simulink model "Controlador_PID_discreto"  (R2021a)
settings: Solver=VariableStepAuto  StartTime=0.0  StopTime=10.0  RelTol=1e-3
undefined symbols (not defined in the file): ba, ksa, ksia, ts
settings Model: Creator=fhlla  LastModifiedBy=fhlla

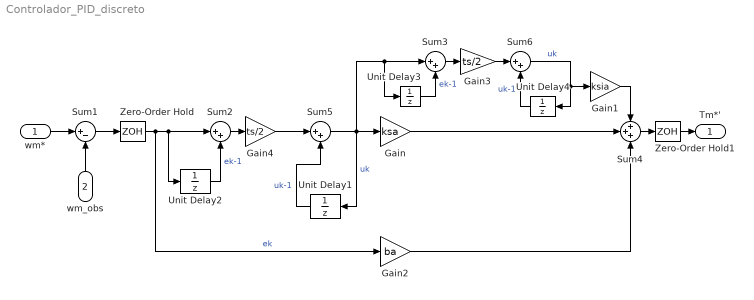
== system Controlador_PID_discreto ==
  wm* : Inport
  wm_obs : Inport  Port=2
  Gain : Gain  Gain=ksa
  Gain1 : Gain  Gain=ksia
  Gain2 : Gain  Gain=ba
  Gain3 : Gain  Gain=ts/2
  Gain4 : Gain  Gain=ts/2
  Sum1 : Sum  Inputs=|+-
  Sum{2..3,5..6} (4 alike) : Sum  Inputs=|++
  Sum4 : Sum  Inputs=+++
  Unit Delay{1..4} (4 alike) : UnitDelay  SampleTime=-1  HasFrameUpgradeWarning=on
  Zero-Order Hold : ZeroOrderHold  SampleTime=-1
  Zero-Order Hold1 : ZeroOrderHold  SampleTime=-1
  Tm*' : Outport
  wires:
  Sum2/1 -> Gain4/1
  Sum5/1 -> Gain/1, Unit Delay3/1, Sum3/1, Unit Delay1/1  "uk"
  Gain3/1 -> Sum6/1
  Sum6/1 -> Gain1/1, Unit Delay4/1  "uk"
  Unit Delay3/1 -> Sum3/2  "ek-1"
  Unit Delay4/1 -> Sum6/2  "uk-1"
  Unit Delay2/1 -> Sum2/2  "ek-1"
  Sum3/1 -> Gain3/1
  Unit Delay1/1 -> Sum5/2  "uk-1"
  Gain4/1 -> Sum5/1
  Gain/1 -> Sum4/2
  Sum4/1 -> Zero-Order Hold1/1
  Zero-Order Hold1/1 -> Tm*'/1
  Gain1/1 -> Sum4/1
  Zero-Order Hold/1 -> Unit Delay2/1, Sum2/1, Gain2/1  "ek"
  wm_obs/1 -> Sum1/2
  Gain2/1 -> Sum4/3
  Sum1/1 -> Zero-Order Hold/1
  wm*/1 -> Sum1/1
